simulink model "fuzzy_control"  (R2022b)
settings: Solver=VariableStepAuto  StartTime=0.0  StopTime=50  RelTol=1e-3
libraries: fuzblock x1
settings Model: Creator=angus  LastModifiedBy=angus

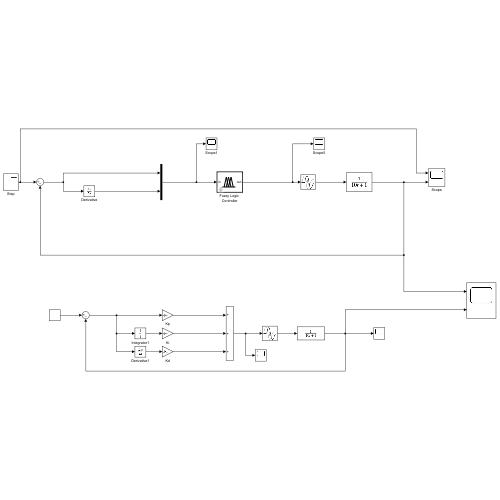
[thumbnail: Simulink's stored preview of the top-level diagram]
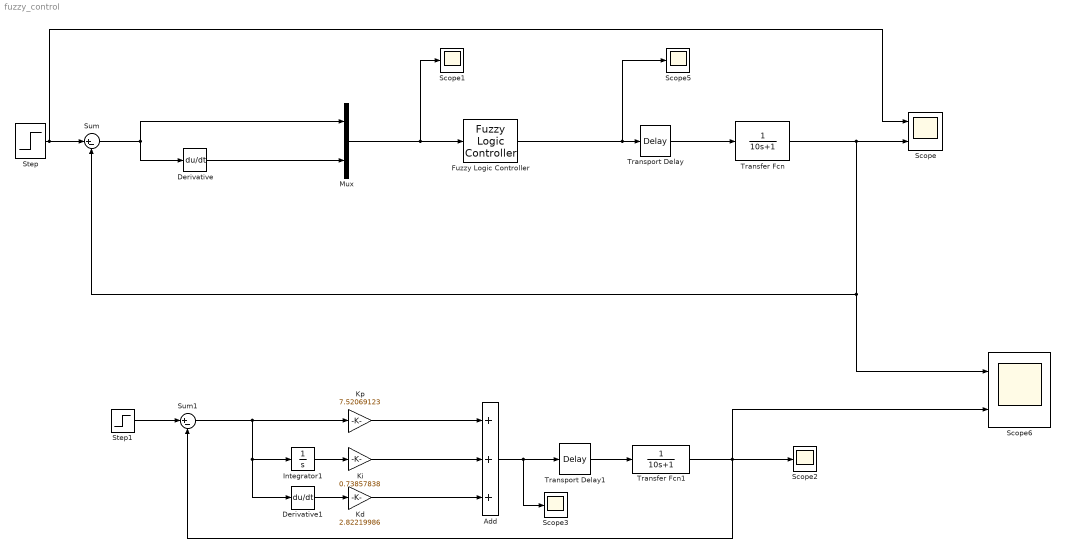
== system fuzzy_control ==
  Add : Sum  Inputs=+++
  Derivative : Derivative
  Derivative1 : Derivative
  Fuzzy Logic Controller : fuzblock/Fuzzy Logic  Controller  FIS=fuzzyrules2  OutputSampleNumber=101  DataType=double  FuzzifiedInputs=off  RuleFiringStrengths=off  RuleOutputs=off  AggregatedOutputs=off  SimulateUsing=Interpreted execution  OutOfRangeInputValueMessage=warning  NoRuleFiredMessage=warning  EmptyOutputFuzzySetMessage=warning
  Integrator1 : Integrator
  Kd : Gain  Gain=2.82219986
  Ki : Gain  Gain=0.73857838
  Kp : Gain  Gain=7.52069123
  Mux : Mux  Inputs=2
  Scope : Scope  NumInputPorts=2
  Scope{1..3,5} (4 alike) : Scope
  Scope6 : Scope  NumInputPorts=2
  Step : Step  SampleTime=0
  Step1 : Step  SampleTime=0
  Sum : Sum  Inputs=|+-
  Sum1 : Sum  Inputs=|+-
  Transfer Fcn : TransferFcn  Denominator=[10 1]
  Transfer Fcn1 : TransferFcn  Denominator=[10 1]
  Transport Delay : TransportDelay
  Transport Delay1 : TransportDelay
  wires:
  Transport Delay/1 -> Transfer Fcn/1
  Mux/1 -> Scope1/1, Fuzzy Logic Controller/1
  Sum/1 -> Mux/1, Derivative/1
  Fuzzy Logic Controller/1 -> Scope5/1, Transport Delay/1
  Derivative/1 -> Mux/2
  Transport Delay1/1 -> Transfer Fcn1/1
  Kd/1 -> Add/3
  Sum1/1 -> Derivative1/1, Integrator1/1, Kp/1
  Step1/1 -> Sum1/1
  Integrator1/1 -> Ki/1
  Derivative1/1 -> Kd/1
  Ki/1 -> Add/2
  Kp/1 -> Add/1
  Transfer Fcn/1 -> Scope6/1, Sum/2, Scope/2
  Add/1 -> Scope3/1, Transport Delay1/1
  Step/1 -> Scope/1, Sum/1
  Transfer Fcn1/1 -> Scope6/2, Sum1/2, Scope2/1
